simulink model "DynamicTemplate"  (R2018b)
settings: Solver=FixedStepDiscrete  StartTime=0.0  StopTime=Inf  FixedStep=0.001  RelTol=1e-3  EnableMultiTasking=on
undefined symbols (not defined in the file): J1, J2, J3, J4, J5, J6, J7, Motor_Current, Motor_Position, Motor_Velocity, Send_GUIdata
libraries: c280xlib x50, simulink x5, idelinklib_common x1
(part 5 of 5)

== stateflow chart DynamicTemplate/DynamicsController/DriverOneMotor/驱动器指令/DriveOder ==
  state State03
    entry:
    MSG=BG
    %开始执行
  state State02
    entry:
    MSG=UM1
    %切换到电流模式
  state State04
    during:
    MSG=TF(Current);
    %电流前馈
  state State01
    entry:
    start=0;
    during:
    start=start_arm(StartRobot)
    %启动机械臂
  state State05
    entry:
    bx=0;
    during:
    bx=check(write)
  state MSG = UM1 [function]
  state MSG = BG [function]
  state MSG = TF(Current) [function]
  state start = start_arm(StartRobot) [function]
  state bx = check(write) [function]
  (default) -> State01
  State02 -> State03 : after(0.5,sec)
  State03 -> State04 : after(0.5,sec)
  State05 -> State02 : [bx>0]
  State01 -> State05 : [start>0]
  data: MSG function_output uint16 size=8; MSG function_output uint16 size=8; Current function_input uint16 size=1; MSG function_output uint16 size=8; StartRobot function_input uint16 size=1; start function_output uint16 size=1; write function_input uint16 size=1; bx function_output uint16 size=1; Current input size=1; MSG output uint16 size=[8 1]; start local uint16; StartRobot input uint16; write input; bx local uint16

== stateflow chart DynamicTemplate/DynamicsController/DriverThreeMotor/驱动器指令/Chart2 ==
  state State03
    entry:
    [MSG1,MSG2,MSG3] = BG
    %开始执行
  state State05
    entry:
    start=0;
    during:
    start=start_arm(StartRobot)
    %启动机械臂
  state State01
    entry:
    bx=0;
    during:
    bx=check(write)
  state State02
    entry:
    [MSG1,MSG2,MSG3] = UM1
    %切换到电流模式
  state State04
    during:
    [MSG1,MSG2,MSG3] = TF(Current1,Current2,Current3)
    %电流前馈
  state bx = check(write) [function]
  state [MSG1,MSG2,MSG3] = UM1 [function]
  state [MSG1,MSG2,MSG3] = BG [function]
  state [MSG1,MSG2,MSG3] = TF(Current1,Current2,Current3) [function]
  state start = start_arm(StartRobot) [function]
  (default) -> State05
  State02 -> State03 : after(0.1,sec)
  State01 -> State02 : [bx>0]
  State03 -> State04 : after(0.1,sec)
  State05 -> State01 : [start>0]
  data: write function_input uint16 size=1; bx function_output uint16 size=1; MSG1 function_output uint16 size=8; MSG2 function_output uint16 size=8; MSG3 function_output uint16 size=8; MSG1 function_output uint16 size=8; MSG2 function_output uint16 size=8; MSG3 function_output uint16 size=8; Current1 function_input uint16 size=1; Current2 function_input uint16 size=1; Current3 function_input uint16 size=1; MSG1 function_output uint16 size=8; MSG2 function_output uint16 size=8; MSG3 function_output uint16 size=8; StartRobot function_input uint16 size=1; start function_output uint16 size=1; write input; MSG1 output uint16 size=8; MSG2 output uint16 size=8; Current1 input; Current2 input; bx local uint16; MSG3 output uint16 size=8; Current3 input; start local uint16; StartRobot input uint16

== stateflow chart DynamicTemplate/DynamicsController/DriverTwoMotor/驱动器指令/Chart2 ==
  state State05
    entry:
    start=0;
    during:
    start=start_arm(StartRobot)
    %启动机械臂
  state State03
    entry:
    [MSG1,MSG2] = BG
    %开始执行
  state State01
    entry:
    bx=0;
    during:
    bx=check(write)
  state State02
    entry:
    [MSG1,MSG2] = UM1
    %切换到电流模式
  state State04
    during:
    [MSG1,MSG2] = TF(Current1,Current2)
    %电流前馈
  state [MSG1,MSG2] = UM1 [function]
  state [MSG1,MSG2] = BG [function]
  state bx = check(write) [function]
  state [MSG1,MSG2] = TF(Current1,Current2) [function]
  state start = start_arm(StartRobot) [function]
  (default) -> State05
  State02 -> State03 : after(0.1,sec)
  State01 -> State02 : [bx>0]
  State03 -> State04 : after(0.1,sec)
  State05 -> State01 : [start>0]
  data: MSG1 function_output uint16 size=8; MSG2 function_output uint16 size=8; MSG1 function_output uint16 size=8; MSG2 function_output uint16 size=8; write function_input uint16 size=1; bx function_output uint16 size=1; MSG1 function_output uint16 size=8; Current1 function_input uint16 size=1; Current2 function_input uint16 size=1; MSG2 function_output uint16 size=8; StartRobot function_input uint16 size=1; start function_output uint16 size=1; MSG1 output uint16 size=8; MSG2 output uint16 size=8; Current1 input; Current2 input; bx local uint16; write input; start local uint16; StartRobot input uint16

== stateflow chart DynamicTemplate/DynamicsController/DriveMotor/驱动器指令/Chart2 ==
  state bx = check(write) [function]
  state MSG = UM1 [function]
  state start = start_arm(StartRobot) [function]
  state State05
    entry:
    start=0;
    during:
    start=start_arm(StartRobot);
    %启动机械臂
  state State01
    entry:
    bx=0;
    during:
    bx=check(write);
  state State06
    entry:
    MSG = UM1;
  state State03
    entry:
    MSG = BG;
  state MSG = TF(Current) [function]
  state State04
    entry:
    during:
    MSG = TF(Current);
  state MSG = BG [function]
  State01 -> State06 : [bx>0]
  (default) -> State05
  State05 -> State01 : [start>0]
  State06 -> State03
  State03 -> State04
  data: write function_input uint16 size=1; bx function_output uint16 size=1; MSG function_output; StartRobot function_input uint16 size=1; start function_output uint16 size=1; MSG function_output; Current function_input uint16 size=[1 6]; MSG function_output; MSG output; Current input size=[1 6]; write input uint16 size=1; bx local uint16 size=1; start local uint16; StartRobot input uint16
